simulink model "SecondaryPath_ANC"  (R2022a)
settings: Solver=FixedStepDiscrete  StartTime=0.0  StopTime=3  FixedStep=0.00025  RelTol=1e-3
libraries: dspadpt3 x1, dspsrcs4 x1
settings Model: Creator=The MathWorks, Inc.  LastModifiedBy=The MathWorks, Inc.
settings SolverCC: AlgebraicLoopSolver=TrustRegion
settings DataIOCC: ReturnWorkspaceOutputs=off
settings DebuggingCC: UnconnectedInputMsg=warning  UnconnectedOutputMsg=warning  UnconnectedLineMsg=warning  SFMachineParentedDataDiag=warning  ArithmeticOperatorsInVariantConditions=warning
settings SFSimCC: CustomCodeUndefinedFunction=UseInterfaceOnly

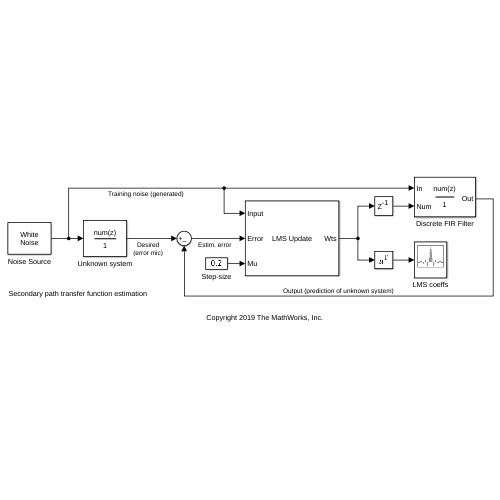
[thumbnail: Simulink's stored preview of the top-level diagram]
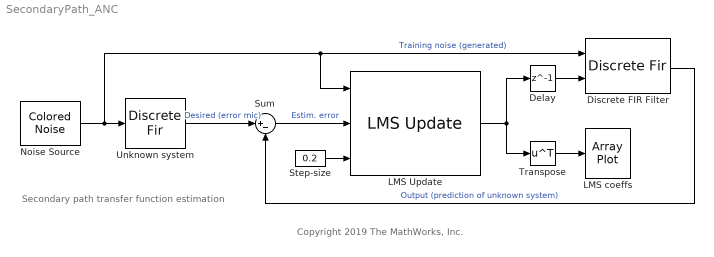
== system SecondaryPath_ANC ==
  note: Copyright 2019 The MathWorks, Inc.
  note: Secondary path transfer function estimation
  Delay : Delay  DelayLength=1
  Discrete FIR Filter : DiscreteFir  CoefSource=Input port
      settings: InputPortMap=u0,u1
  LMS Update : dspadpt3/LMS Update  Method=Normalized LMS  Length=32  NumFilters=1  StepSizeSource=Input port  StepSize=0.1  LeakageFactor=1.0  InitialConditions=0  AdaptiveFilterMode=Tapped delay-line FIR filter  EnableAdaptInput=off  EnableResetInput=off  SimulateUsing=Interpreted execution
      settings: SourceProductBaseCode=DS
  LMS coeffs : ArrayPlot  WindowPosition=[233.000000,288.000000,800.000000,500.000000,]  Visible=on  ScopeFrameLocation=window  AxesScaling=Manual  YLimits=[-0.624999,0.624999]  DefaultConfigurationName=dsp.scopes.ArrayPlotBlockSpecification
  Noise Source : dspsrcs4/Colored Noise  Color=white  InverseFrequencyPower=1  BoundedOutput=off  NumChannels=1  OutputDataType=double  SamplesPerFrame=1  SampleTime=1/4000  RandomStream=mt19937ar with seed  Seed=67  SimulateUsing=Interpreted execution
      settings: SourceProductBaseCode=DS
  Step-size : Constant  Value=0.2
  Sum : Sum  Inputs=|+-
  Transpose : Math  Operator=transpose  SignedPower=on
  Unknown system : DiscreteFir  Coefficients=[0 0 -.5 .5 -.3 .2 -.1 .5 -.5]  InputProcessing=Columns as channels (frame based)
  wires:
  Transpose/1 -> LMS coeffs/1
  Step-size/1 -> LMS Update/3
  Unknown system/1 -> Sum/1  "Desired (error mic)"
  Sum/1 -> LMS Update/2  "Estim. error"
  Discrete FIR Filter/1 -> Sum/2  "Output (prediction of unknown system)"
  Noise Source/1 -> LMS Update/1, Discrete FIR Filter/1, Unknown system/1  "Training noise (generated)"
  LMS Update/1 -> Transpose/1, Delay/1
  Delay/1 -> Discrete FIR Filter/2
